simulink model "plant"  (R2024b)
settings: Solver=VariableStepAuto  StartTime=0.0  StopTime=10.0  RelTol=1e-3
values from neighbouring files (symbols this model uses):
  X_air = evalin('base', 'X_air')    [init_fn.m]
undefined symbols (not defined in the file or in its folder): m, MAX_SPEED_BACKWARD, MAX_SPEED_FORWARD, r, TRANSMISSION_RATIO, X_tyres
settings Model: Creator=DAUIN-Win10  LastModifiedBy=aayan
settings OptimizationCC: ReuseModelBlockBuffer=off
settings DebuggingCC: UnconnectedInputMsg=warning  UnconnectedOutputMsg=warning  UnconnectedLineMsg=warning
settings ModelReferenceCC: EnableRefExpFcnMdlSchedulingChecks=on
settings RTWCC: GPUComputeCapability=3.5  DLArmComputeVersion=19.05

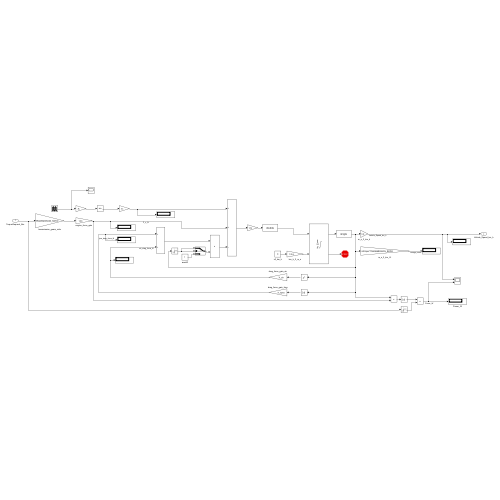
[thumbnail: Simulink's stored preview of the top-level diagram]
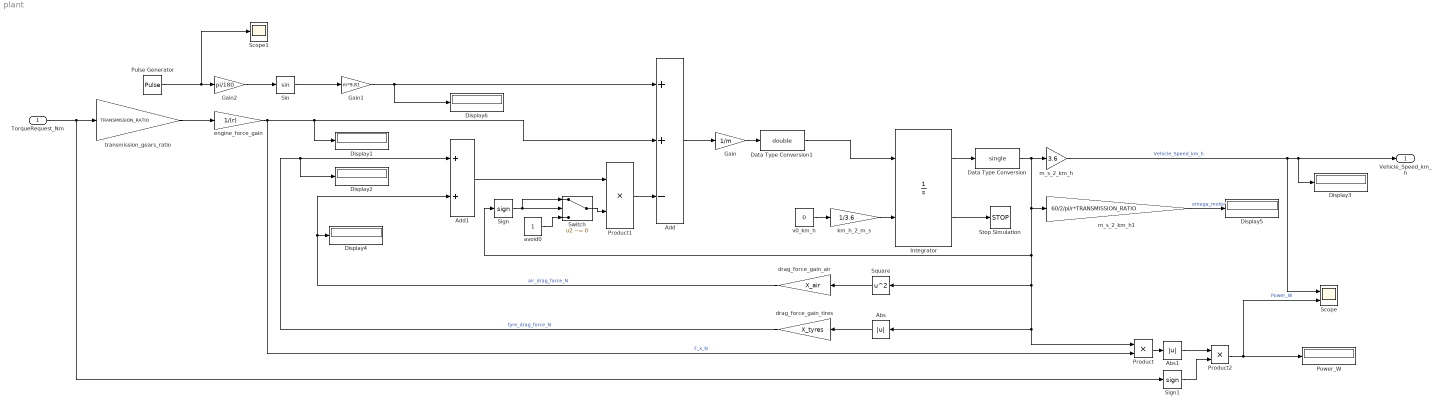
== system plant ==
  TorqueRequest_Nm : Inport  OutDataTypeStr=single
  Abs : Abs  SaturateOnIntegerOverflow=off
  Abs1 : Abs  SaturateOnIntegerOverflow=off
  Add : Sum  Inputs=++-
  Add1 : Sum
  Data Type Conversion : DataTypeConversion  OutDataTypeStr=single  SaturateOnIntegerOverflow=off  RndMeth=Floor  LockScale=on
  Data Type Conversion1 : DataTypeConversion  OutDataTypeStr=double  SaturateOnIntegerOverflow=off  RndMeth=Floor  LockScale=on
  Display{1..6} (6 alike) : Display
      settings: Format=bank
  Gain : Gain  Gain=1/m
  Gain1 : Gain  Gain=m*9.81
  Gain2 : Gain  Gain=pi/180
  Integrator : Integrator  InitialConditionSource=external  LimitOutput=on  UpperSaturationLimit=MAX_SPEED_FORWARD/3.6  LowerSaturationLimit=-MAX_SPEED_BACKWARD/3.6  ShowSaturationPort=on  ContinuousStateAttributes='vehicle_speed'
  Power_W : Display
      settings: Format=bank
  Product : Product
  Product1 : Product
  Product2 : Product
  Pulse Generator : DiscretePulseGenerator  PulseType=Time based  Amplitude=0  PulseWidth=50  PhaseDelay=5
  Scope : Scope  NumInputPorts=2
  Scope1 : Scope
  Sign : Signum  ZeroCross=off
  Sign1 : Signum  ZeroCross=off
  Sin : Trigonometry  OutputSignalType=real
  Square : Math  Operator=square
  Stop Simulation : Stop
  Switch : Switch  Criteria=u2 ~= 0  SaturateOnIntegerOverflow=off  InputSameDT=off
  avoid0 : Constant  OutDataTypeStr=double
  drag_force_gain_air : Gain  Gain=X_air
  drag_force_gain_tires : Gain  Gain=X_tyres
  engine_force_gain : Gain  Gain=1/(r)
  km_h_2_m_s : Gain  Gain=1/3.6
  m_s_2_km_h : Gain  Gain=3.6
  m_s_2_km_h1 : Gain  Gain=60/2/pi/r*TRANSMISSION_RATIO
  transmission_gears_ratio : Gain  Gain=TRANSMISSION_RATIO
  v0_km_h : Constant  Value=0  OutDataTypeStr=double
  Vehicle_Speed_km_h : Outport  OutDataTypeStr=single  Unit=km/h
  wires:
  v0_km_h/1 -> km_h_2_m_s/1
  km_h_2_m_s/1 -> Integrator/2
  TorqueRequest_Nm/1 -> Sign1/1, transmission_gears_ratio/1
  Data Type Conversion/1 -> Sign/1, Product/1, Abs/1, Square/1, m_s_2_km_h1/1, m_s_2_km_h/1
  Integrator/1 -> Data Type Conversion/1
  transmission_gears_ratio/1 -> engine_force_gain/1
  engine_force_gain/1 -> Product/2, Display1/1, Add/2  "F_x_N"
  m_s_2_km_h/1 -> Vehicle_Speed_km_h/1, Display3/1, Scope/1  "Vehicle_Speed_km_h"
  Square/1 -> drag_force_gain_air/1
  drag_force_gain_air/1 -> Add1/2, Display4/1  "air_drag_force_N"
  Gain/1 -> Data Type Conversion1/1
  drag_force_gain_tires/1 -> Display2/1, Add1/1  "tyre_drag_force_N"
  m_s_2_km_h1/1 -> Display5/1  "omega_motor"
  Integrator/2 -> Stop Simulation/1
  Add/1 -> Gain/1
  Sign/1 -> Switch/1, Switch/2
  avoid0/1 -> Switch/3
  Abs/1 -> drag_force_gain_tires/1
  Product2/1 -> Scope/2, Power_W/1  "Power_W"
  Product/1 -> Abs1/1
  Sign1/1 -> Product2/2
  Abs1/1 -> Product2/1
  Sin/1 -> Gain1/1
  Gain1/1 -> Display6/1, Add/1
  Gain2/1 -> Sin/1
  Pulse Generator/1 -> Scope1/1, Gain2/1
  Switch/1 -> Product1/2
  Data Type Conversion1/1 -> Integrator/1
  Add1/1 -> Product1/1
  Product1/1 -> Add/3
